simulink subsystem "HI_FastAnalogInputs"  (R2019b)
settings: Solver=VariableStepAuto  StartTime=0.0  StopTime=10.0  RelTol=1e-3
libraries: c2802xlib x4
settings Model: Creator=Nick  LastModifiedBy=Nick

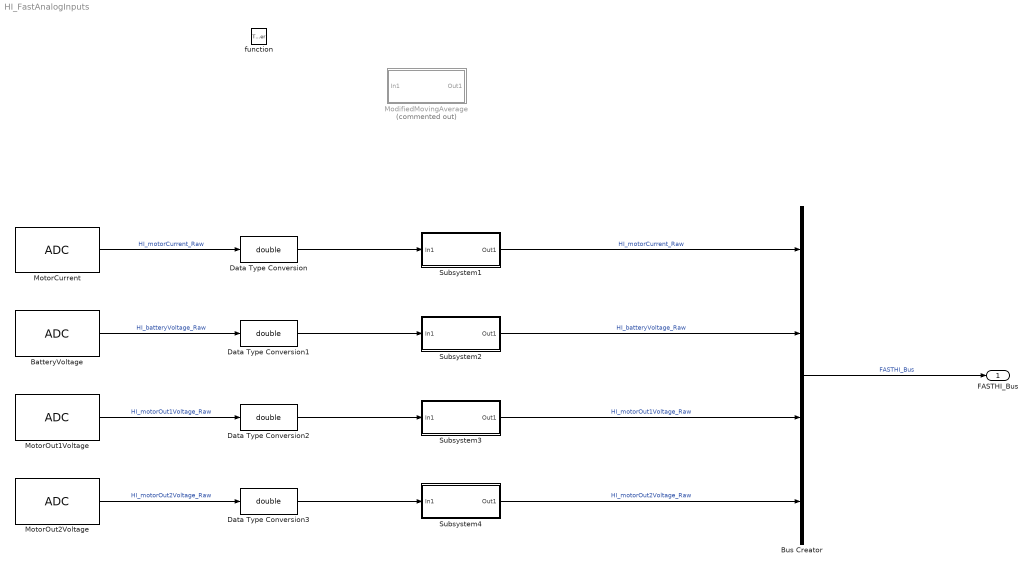
== system HI_FastAnalogInputs ==
  function : TriggerPort  TriggerType=function-call  VariantControl=Variant
  BatteryVoltage : c2802xlib/ADC  blkParamProc=C2000_Type4  ADCModule=B  samplingMode=Single sample mode  ADCResolution=12-bit (Single-ended input)  useSOC1=SOC3  useSOC2=SOC0_SOC1  SOCAcquisitionWindow=15  SOCTriggerSource=Software  SOCInterruptTrigger=No ADCINT  Ts=-1  dType=uint16  postInterrupt=off  interruptSel=ADCINT1  ADCINTContinuous=on  endma=off  chdma=1  conv1=ADCINA0  conv2=ADCINA0 and ADCINB0  conv1_Type4=ADCIN14  conv2_Type4=ADCIN0 and ADCIN1
      settings: SourceProductName=Embedded Coder Support Package for Texas Instruments C2000 Processors
  Bus Creator : BusCreator  Inputs=4
  Data Type Conversion{,1..3} (4 alike) : DataTypeConversion  OutDataTypeStr=double
  ModifiedMovingAverage : Subsystem  Commented=on
  MotorCurrent : c2802xlib/ADC  blkParamProc=C2000_Type4  ADCModule=B  samplingMode=Single sample mode  ADCResolution=12-bit (Single-ended input)  useSOC1=SOC2  useSOC2=SOC0_SOC1  SOCAcquisitionWindow=15  SOCTriggerSource=Software  SOCInterruptTrigger=No ADCINT  Ts=-1  dType=uint16  postInterrupt=off  interruptSel=ADCINT1  ADCINTContinuous=on  endma=off  chdma=1  conv1=ADCINA0  conv2=ADCINA0 and ADCINB0  conv1_Type4=ADCIN4  conv2_Type4=ADCIN0 and ADCIN1
      settings: SourceProductName=Embedded Coder Support Package for Texas Instruments C2000 Processors
  MotorOut1Voltage : c2802xlib/ADC  blkParamProc=C2000_Type4  ADCModule=B  samplingMode=Single sample mode  ADCResolution=12-bit (Single-ended input)  useSOC1=SOC0  useSOC2=SOC0_SOC1  SOCAcquisitionWindow=15  SOCTriggerSource=Software  SOCInterruptTrigger=No ADCINT  Ts=-1  dType=uint16  postInterrupt=off  interruptSel=ADCINT1  ADCINTContinuous=on  endma=off  chdma=1  conv1=ADCINA0  conv2=ADCINA0 and ADCINB0  conv1_Type4=ADCIN2  conv2_Type4=ADCIN0 and ADCIN1
      settings: SourceProductName=Embedded Coder Support Package for Texas Instruments C2000 Processors
  MotorOut2Voltage : c2802xlib/ADC  blkParamProc=C2000_Type4  ADCModule=B  samplingMode=Single sample mode  ADCResolution=12-bit (Single-ended input)  useSOC1=SOC1  useSOC2=SOC0_SOC1  SOCAcquisitionWindow=15  SOCTriggerSource=Software  SOCInterruptTrigger=No ADCINT  Ts=-1  dType=uint16  postInterrupt=off  interruptSel=ADCINT1  ADCINTContinuous=on  endma=off  chdma=1  conv1=ADCINA0  conv2=ADCINA0 and ADCINB0  conv1_Type4=ADCIN1  conv2_Type4=ADCIN0 and ADCIN1
      settings: SourceProductName=Embedded Coder Support Package for Texas Instruments C2000 Processors
  Subsystem1 : Subsystem
  Subsystem2 : Subsystem
  Subsystem3 : Subsystem
  Subsystem4 : Subsystem
  FASTHI_Bus : Outport
  wires:
  Bus Creator/1 -> FASTHI_Bus/1  "FASTHI_Bus"
  MotorOut2Voltage/1 -> Data Type Conversion3/1  "HI_motorOut2Voltage_Raw"
  MotorOut1Voltage/1 -> Data Type Conversion2/1  "HI_motorOut1Voltage_Raw"
  BatteryVoltage/1 -> Data Type Conversion1/1  "HI_batteryVoltage_Raw"
  MotorCurrent/1 -> Data Type Conversion/1  "HI_motorCurrent_Raw"
  Subsystem1/1(Out1) -> Bus Creator/1  "HI_motorCurrent_Raw"
  Subsystem2/1(Out1) -> Bus Creator/2  "HI_batteryVoltage_Raw"
  Subsystem3/1(Out1) -> Bus Creator/3  "HI_motorOut1Voltage_Raw"
  Subsystem4/1(Out1) -> Bus Creator/4  "HI_motorOut2Voltage_Raw"
  Data Type Conversion/1 -> Subsystem1/1(In1)
  Data Type Conversion1/1 -> Subsystem2/1(In1)
  Data Type Conversion2/1 -> Subsystem3/1(In1)
  Data Type Conversion3/1 -> Subsystem4/1(In1)

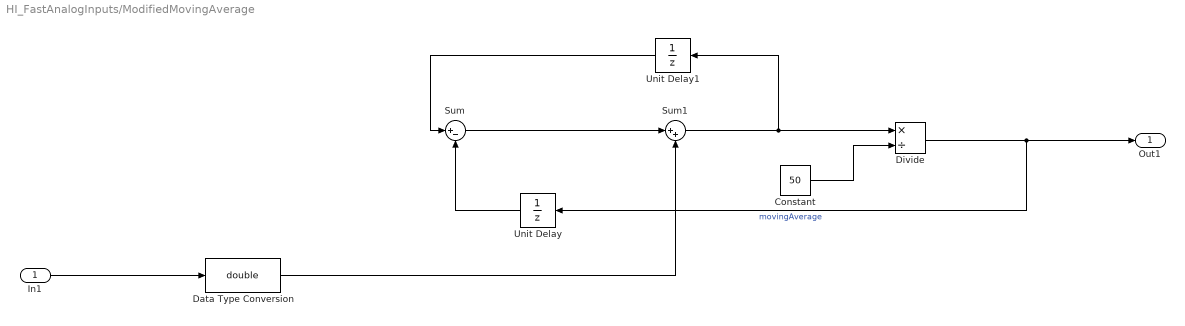
== system HI_FastAnalogInputs/ModifiedMovingAverage ==
  In1 : Inport
  Constant : Constant  Value=50
  Data Type Conversion : DataTypeConversion  OutDataTypeStr=double
  Divide : Product  Inputs=*/
  Sum : Sum  Inputs=|+-
  Sum1 : Sum  Inputs=|++
  Unit Delay : UnitDelay  SampleTime=-1  HasFrameUpgradeWarning=on
  Unit Delay1 : UnitDelay  SampleTime=-1  HasFrameUpgradeWarning=on
  Out1 : Outport
  wires:
  Unit Delay/1 -> Sum/2
  Unit Delay1/1 -> Sum/1
  Divide/1 -> Out1/1, Unit Delay/1  "movingAverage"
  Constant/1 -> Divide/2
  Sum1/1 -> Divide/1, Unit Delay1/1
  Sum/1 -> Sum1/1
  Data Type Conversion/1 -> Sum1/2
  In1/1 -> Data Type Conversion/1

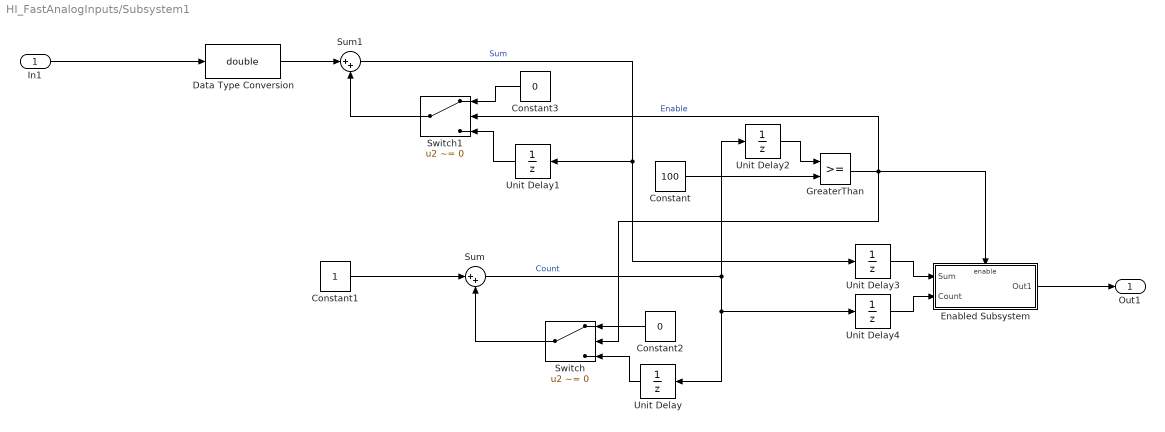
== system HI_FastAnalogInputs/Subsystem1 ==
  In1 : Inport
  Constant : Constant  Value=100
  Constant1 : Constant
  Constant2 : Constant  Value=0
  Constant3 : Constant  Value=0
  Data Type Conversion : DataTypeConversion  OutDataTypeStr=double
  Enabled Subsystem : Subsystem  TreatAsAtomicUnit=on
  GreaterThan : RelationalOperator  OutDataTypeStr=boolean  RndMeth=Simplest
  Sum : Sum  Inputs=|++
  Sum1 : Sum  Inputs=|++
  Switch : Switch  Criteria=u2 ~= 0  Threshold=50
  Switch1 : Switch  Criteria=u2 ~= 0  Threshold=50
  Unit Delay{,1..4} (5 alike) : UnitDelay  SampleTime=-1  HasFrameUpgradeWarning=on
  Out1 : Outport
  wires:
  Unit Delay3/1 -> Enabled Subsystem/1(Sum)
  Unit Delay4/1 -> Enabled Subsystem/2(Count)
  Unit Delay2/1 -> GreaterThan/1
  Switch1/1 -> Sum1/2
  Constant3/1 -> Switch1/1
  Unit Delay1/1 -> Switch1/3
  Data Type Conversion/1 -> Sum1/1
  Switch/1 -> Sum/2
  Constant2/1 -> Switch/1
  Unit Delay/1 -> Switch/3
  Constant1/1 -> Sum/1
  GreaterThan/1 -> Enabled Subsystem/Enable, Switch/2, Switch1/2  "Enable"
  Sum/1 -> Unit Delay2/1, Unit Delay/1, Unit Delay4/1  "Count"
  Sum1/1 -> Unit Delay1/1, Unit Delay3/1  "Sum"
  Constant/1 -> GreaterThan/2
  Enabled Subsystem/1(Out1) -> Out1/1
  In1/1 -> Data Type Conversion/1

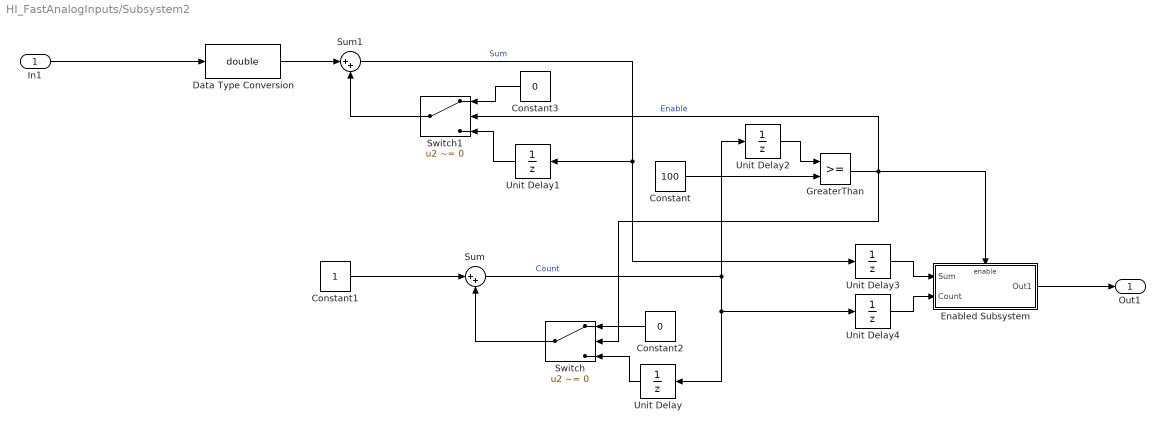
== system HI_FastAnalogInputs/Subsystem2 ==
  In1 : Inport
  Constant : Constant  Value=100
  Constant1 : Constant
  Constant2 : Constant  Value=0
  Constant3 : Constant  Value=0
  Data Type Conversion : DataTypeConversion  OutDataTypeStr=double
  Enabled Subsystem : Subsystem  TreatAsAtomicUnit=on
  GreaterThan : RelationalOperator  OutDataTypeStr=boolean  RndMeth=Simplest
  Sum : Sum  Inputs=|++
  Sum1 : Sum  Inputs=|++
  Switch : Switch  Criteria=u2 ~= 0  Threshold=50
  Switch1 : Switch  Criteria=u2 ~= 0  Threshold=50
  Unit Delay{,1..4} (5 alike) : UnitDelay  SampleTime=-1  HasFrameUpgradeWarning=on
  Out1 : Outport
  wires:
  Unit Delay3/1 -> Enabled Subsystem/1(Sum)
  Unit Delay4/1 -> Enabled Subsystem/2(Count)
  Unit Delay2/1 -> GreaterThan/1
  Switch1/1 -> Sum1/2
  Constant3/1 -> Switch1/1
  Unit Delay1/1 -> Switch1/3
  Data Type Conversion/1 -> Sum1/1
  Switch/1 -> Sum/2
  Constant2/1 -> Switch/1
  Unit Delay/1 -> Switch/3
  Constant1/1 -> Sum/1
  GreaterThan/1 -> Enabled Subsystem/Enable, Switch/2, Switch1/2  "Enable"
  Sum/1 -> Unit Delay2/1, Unit Delay/1, Unit Delay4/1  "Count"
  Sum1/1 -> Unit Delay1/1, Unit Delay3/1  "Sum"
  Constant/1 -> GreaterThan/2
  Enabled Subsystem/1(Out1) -> Out1/1
  In1/1 -> Data Type Conversion/1

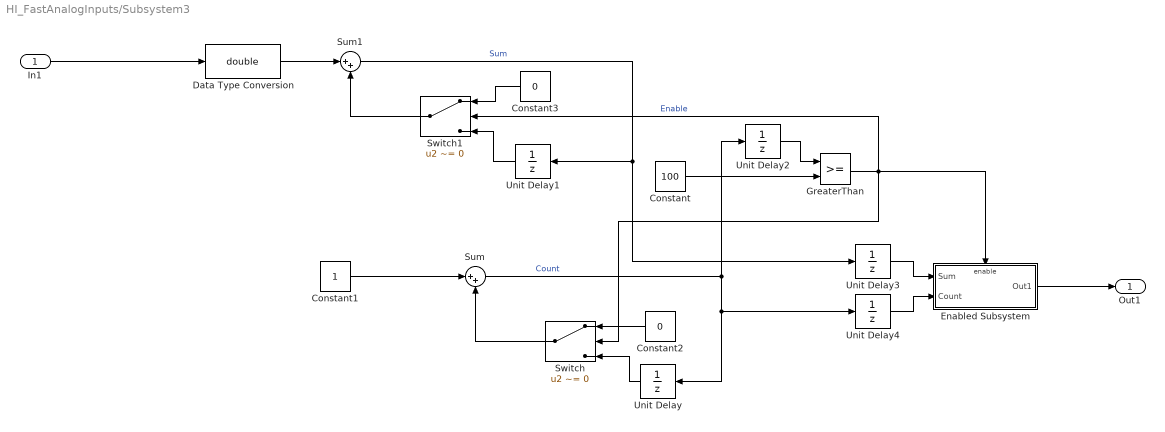
== system HI_FastAnalogInputs/Subsystem3 ==
  In1 : Inport
  Constant : Constant  Value=100
  Constant1 : Constant
  Constant2 : Constant  Value=0
  Constant3 : Constant  Value=0
  Data Type Conversion : DataTypeConversion  OutDataTypeStr=double
  Enabled Subsystem : Subsystem  TreatAsAtomicUnit=on
  GreaterThan : RelationalOperator  OutDataTypeStr=boolean  RndMeth=Simplest
  Sum : Sum  Inputs=|++
  Sum1 : Sum  Inputs=|++
  Switch : Switch  Criteria=u2 ~= 0  Threshold=50
  Switch1 : Switch  Criteria=u2 ~= 0  Threshold=50
  Unit Delay{,1..4} (5 alike) : UnitDelay  SampleTime=-1  HasFrameUpgradeWarning=on
  Out1 : Outport
  wires:
  Unit Delay3/1 -> Enabled Subsystem/1(Sum)
  Unit Delay4/1 -> Enabled Subsystem/2(Count)
  Unit Delay2/1 -> GreaterThan/1
  Switch1/1 -> Sum1/2
  Constant3/1 -> Switch1/1
  Unit Delay1/1 -> Switch1/3
  Data Type Conversion/1 -> Sum1/1
  Switch/1 -> Sum/2
  Constant2/1 -> Switch/1
  Unit Delay/1 -> Switch/3
  Constant1/1 -> Sum/1
  GreaterThan/1 -> Enabled Subsystem/Enable, Switch/2, Switch1/2  "Enable"
  Sum/1 -> Unit Delay2/1, Unit Delay/1, Unit Delay4/1  "Count"
  Sum1/1 -> Unit Delay1/1, Unit Delay3/1  "Sum"
  Constant/1 -> GreaterThan/2
  Enabled Subsystem/1(Out1) -> Out1/1
  In1/1 -> Data Type Conversion/1

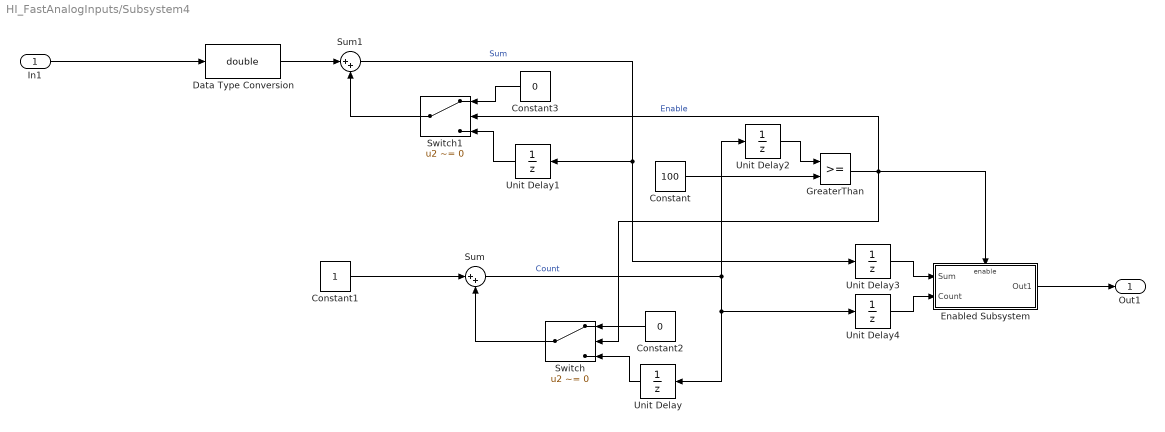
== system HI_FastAnalogInputs/Subsystem4 ==
  In1 : Inport
  Constant : Constant  Value=100
  Constant1 : Constant
  Constant2 : Constant  Value=0
  Constant3 : Constant  Value=0
  Data Type Conversion : DataTypeConversion  OutDataTypeStr=double
  Enabled Subsystem : Subsystem  TreatAsAtomicUnit=on
  GreaterThan : RelationalOperator  OutDataTypeStr=boolean  RndMeth=Simplest
  Sum : Sum  Inputs=|++
  Sum1 : Sum  Inputs=|++
  Switch : Switch  Criteria=u2 ~= 0  Threshold=50
  Switch1 : Switch  Criteria=u2 ~= 0  Threshold=50
  Unit Delay{,1..4} (5 alike) : UnitDelay  SampleTime=-1  HasFrameUpgradeWarning=on
  Out1 : Outport
  wires:
  Unit Delay3/1 -> Enabled Subsystem/1(Sum)
  Unit Delay4/1 -> Enabled Subsystem/2(Count)
  Unit Delay2/1 -> GreaterThan/1
  Switch1/1 -> Sum1/2
  Constant3/1 -> Switch1/1
  Unit Delay1/1 -> Switch1/3
  Data Type Conversion/1 -> Sum1/1
  Switch/1 -> Sum/2
  Constant2/1 -> Switch/1
  Unit Delay/1 -> Switch/3
  Constant1/1 -> Sum/1
  GreaterThan/1 -> Enabled Subsystem/Enable, Switch/2, Switch1/2  "Enable"
  Sum/1 -> Unit Delay2/1, Unit Delay/1, Unit Delay4/1  "Count"
  Sum1/1 -> Unit Delay1/1, Unit Delay3/1  "Sum"
  Constant/1 -> GreaterThan/2
  Enabled Subsystem/1(Out1) -> Out1/1
  In1/1 -> Data Type Conversion/1

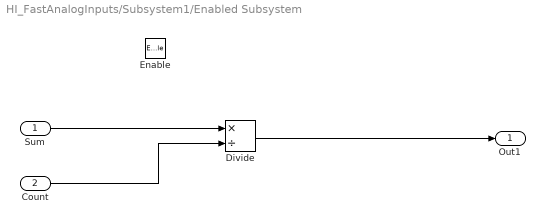
== system HI_FastAnalogInputs/Subsystem1/Enabled Subsystem ==
  Sum : Inport
  Count : Inport  Port=2
  Enable : EnablePort
  Divide : Product  Inputs=*/
  Out1 : Outport
  wires:
  Divide/1 -> Out1/1
  Count/1 -> Divide/2
  Sum/1 -> Divide/1

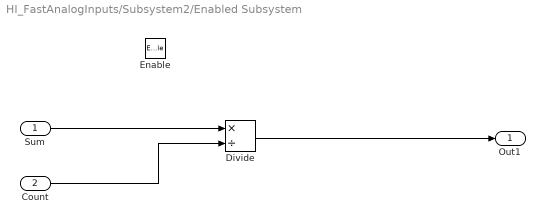
== system HI_FastAnalogInputs/Subsystem2/Enabled Subsystem ==
  Sum : Inport
  Count : Inport  Port=2
  Enable : EnablePort
  Divide : Product  Inputs=*/
  Out1 : Outport
  wires:
  Divide/1 -> Out1/1
  Count/1 -> Divide/2
  Sum/1 -> Divide/1

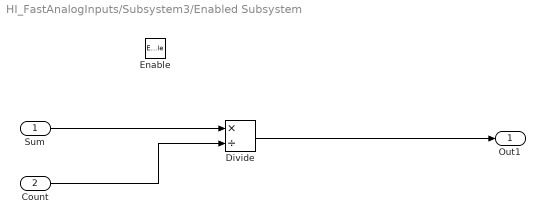
== system HI_FastAnalogInputs/Subsystem3/Enabled Subsystem ==
  Sum : Inport
  Count : Inport  Port=2
  Enable : EnablePort
  Divide : Product  Inputs=*/
  Out1 : Outport
  wires:
  Divide/1 -> Out1/1
  Count/1 -> Divide/2
  Sum/1 -> Divide/1

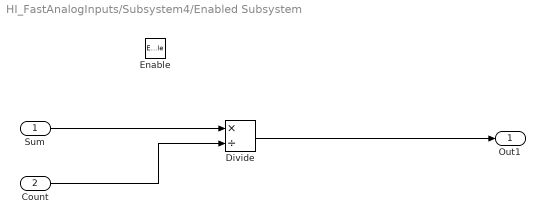
== system HI_FastAnalogInputs/Subsystem4/Enabled Subsystem ==
  Sum : Inport
  Count : Inport  Port=2
  Enable : EnablePort
  Divide : Product  Inputs=*/
  Out1 : Outport
  wires:
  Divide/1 -> Out1/1
  Count/1 -> Divide/2
  Sum/1 -> Divide/1
